simulink model "mdl_closed_loop_mpc"  (R2025a)
settings: Solver=VariableStepAuto  StartTime=0.0  StopTime=40  RelTol=1e-3
undefined symbols (not defined in the file or in its folder): coreData, onlineData
settings Model: Creator=hoshino  LastModifiedBy=root
settings ModelReferenceCC: EnableRefExpFcnMdlSchedulingChecks=on
settings RTWCC: GPUComputeCapability=3.5

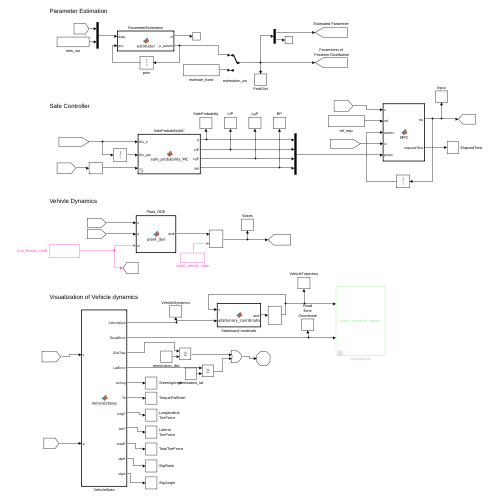
[thumbnail: Simulink's stored preview of the top-level diagram]
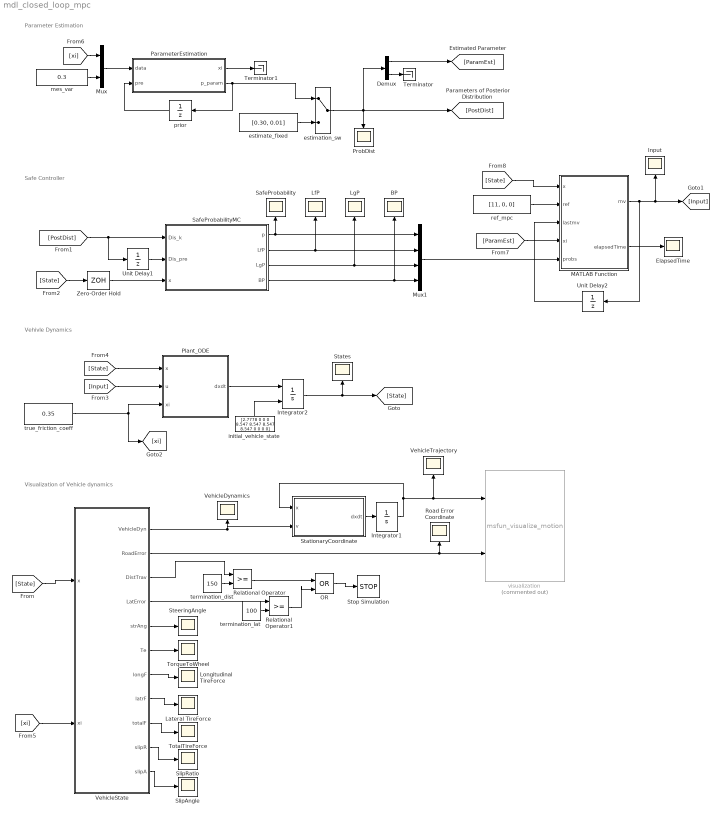
== system mdl_closed_loop_mpc ==
  note: Visualization of Vehicle dynamics
  note: Parameter Estimation
  note: Safe Controller
  note: Vehivle Dynamics
  BP : Scope
      settings: ActiveDisplayYMinimum=-0.13375  ActiveDisplayYMaximum=0.10375  DataLoggingVariableName=BP
  Demux : Demux  Outputs=2
  ElapsedTime : Scope
      settings: SampleTime=0.1  ActiveDisplayYMinimum=-0.96659  ActiveDisplayYMaximum=0.91637  DataLoggingVariableName=ElapsedTime
  Input : Scope
      settings: ActiveDisplayYMinimum=-0.96659  ActiveDisplayYMaximum=0.91637  DataLoggingVariableName=Input
  Integrator1 : Integrator  InitialCondition=[0; 0; 0]
  Integrator2 : Integrator  InitialConditionSource=external
  Lateral TireForce : Scope
      settings: ActiveDisplayYMinimum=-924.98438  ActiveDisplayYMaximum=1900.60095
  LfP : Scope
      settings: ActiveDisplayYMinimum=-5.7375  ActiveDisplayYMaximum=1.6375  DataLoggingVariableName=LfP
  LgP : Scope
      settings: ActiveDisplayYMinimum=-2.175  ActiveDisplayYMaximum=0.575  DataLoggingVariableName=LgP
  Longitudinal TireForce : Scope
      settings: ActiveDisplayYMinimum=-313.11882  ActiveDisplayYMaximum=375.42257
  MATLAB Function : MATLAB Function  TreatAsAtomicUnit=on
  Mux : Mux  Inputs=2
  Mux1 : Mux
  OR : Logic  Operator=OR  IconShape=distinctive  AllPortsSameDT=off  OutDataTypeStr=boolean
  ParameterEstimation : MATLAB Function  TreatAsAtomicUnit=on
  Plant_ODE : MATLAB Function  TreatAsAtomicUnit=on
  ProbDist : Scope
      settings: ActiveDisplayYMinimum=-0.11139  ActiveDisplayYMaximum=1.00583  DataLoggingVariableName=ProbDist
  Relational Operator : RelationalOperator  OutDataTypeStr=boolean  RndMeth=Simplest  InputSameDT=off
  Relational Operator1 : RelationalOperator  OutDataTypeStr=boolean  RndMeth=Simplest  InputSameDT=off
  Road Error Coordinate : Scope
      settings: ActiveDisplayYMinimum=-5E-5  ActiveDisplayYMaximum=0.0002  DataLoggingVariableName=ScopeData3
  SafeProbability : Scope
      settings: ActiveDisplayYMinimum=-0.125  ActiveDisplayYMaximum=1.125  DataLoggingVariableName=SafeProb
  SafeProbabilityMC : MATLAB Function  TreatAsAtomicUnit=on  mask{snum=100, dt=1.5, horizon=5, emax=10}
  SlipAngle : Scope
      settings: ActiveDisplayYMinimum=-0.25893  ActiveDisplayYMaximum=0.1231  DataLoggingVariableName=slipA
  SlipRatio : Scope
      settings: ActiveDisplayYMinimum=-0.0048  ActiveDisplayYMaximum=0.00922  DataLoggingVariableName=slipR
  States : Scope
      settings: SampleTime=0.1  ActiveDisplayYMinimum=-179.2878  ActiveDisplayYMaximum=230.07424  DataLoggingVariableName=State
  StationaryCoordinate : MATLAB Function  TreatAsAtomicUnit=on
  SteeringAngle : Scope
      settings: ActiveDisplayYMinimum=-0.32134275248447025  ActiveDisplayYMaximum=0.39116625122994469
  Stop Simulation : Stop
  Terminator : Terminator
  Terminator1 : Terminator
  TorqueToWheel : Scope
      settings: ActiveDisplayYMinimum=-256.25579  ActiveDisplayYMaximum=271.06293  DataLoggingVariableName=ScopeData2
  TotalTireForce : Scope
      settings: ActiveDisplayYMinimum=-70.03908  ActiveDisplayYMaximum=630.35171  DataLoggingVariableName=TireForce
  Unit Delay1 : UnitDelay  SampleTime=-1  HasFrameUpgradeWarning=on
  Unit Delay2 : UnitDelay  SampleTime=-1  HasFrameUpgradeWarning=on
  VehicleDynamics : Scope
      settings: ActiveDisplayYMinimum=-0.80591  ActiveDisplayYMaximum=6.57776  DataLoggingVariableName=ScopeData2
  VehicleState : MATLAB Function  TreatAsAtomicUnit=on
  VehicleTrajectory : Scope
      settings: SampleTime=0.1  ActiveDisplayYMinimum=81.20316  ActiveDisplayYMaximum=88.79585  DataLoggingVariableName=Trajectory
  Zero-Order Hold : ZeroOrderHold  SampleTime=0.1
  estimate_fixed : Constant  Value=[0.30, 0.01]
  estimation_sw : ManualSwitch
  initial_vehicle_state : Constant  Value="[2.7778           0           0           0       8.547       8.547       8.547       8.547           0           0           0           0]"
  mes_var : Constant  Value=0.3
  prior : UnitDelay  InitialCondition=[0.9 0.3]  SampleTime=-1  HasFrameUpgradeWarning=on
  ref_mpc : Constant  Value=[11, 0, 0]  VectorParams1D=off
  termination_dist : Constant  Value=150
  termination_lat : Constant  Value=100
  true_friction_coeff : Constant  Value=0.35
  visualization : M-S-Function  Commented=on  FunctionName=msfun_visualize_motion
  wires:
  Integrator2/1 -> States/1, [State]
  VehicleState/1(VehicleDyn) -> StationaryCoordinate/2(v), VehicleDynamics/1
  Integrator1/1 -> VehicleTrajectory/1, visualization/1, StationaryCoordinate/1(x)
  StationaryCoordinate/1(dxdt) -> Integrator1/1
  Plant_ODE/1(dxdt) -> Integrator2/1
  initial_vehicle_state/1 -> Integrator2/2
  true_friction_coeff/1 -> Plant_ODE/3(xi), [xi]
  [State] -> VehicleState/1(x)
  MATLAB Function/1(mv) -> Unit Delay2/1, Input/1, [Input]
  ParameterEstimation/2(p_param) -> estimation_sw/1, prior/1
  prior/1 -> ParameterEstimation/2(pre)
  ParameterEstimation/1(xi) -> Terminator1/1
  [State] -> Zero-Order Hold/1
  SafeProbabilityMC/1(p) -> SafeProbability/1, Mux1/1
  Zero-Order Hold/1 -> SafeProbabilityMC/3(x)
  [Input] -> Plant_ODE/2(u)
  [State] -> Plant_ODE/1(x)
  VehicleState/7(longF) -> Longitudinal TireForce/1
  SafeProbabilityMC/4(BP) -> Mux1/4, BP/1
  [PostDist] -> Unit Delay1/1, SafeProbabilityMC/1(Dis_k)
  Unit Delay1/1 -> SafeProbabilityMC/2(Dis_pre)
  VehicleState/9(totalF) -> TotalTireForce/1
  SafeProbabilityMC/2(LfP) -> LfP/1, Mux1/2
  SafeProbabilityMC/3(LgP) -> LgP/1, Mux1/3
  VehicleState/8(latrF) -> Lateral TireForce/1
  [xi] -> VehicleState/2(xi)
  VehicleState/10(slipR) -> SlipRatio/1
  VehicleState/11(slipA) -> SlipAngle/1
  VehicleState/2(RoadError) -> visualization/2, Road Error Coordinate/1
  Mux/1 -> ParameterEstimation/1(data)
  VehicleState/5(strAng) -> SteeringAngle/1
  VehicleState/6(Te) -> TorqueToWheel/1
  Relational Operator/1 -> OR/1
  VehicleState/3(DistTrav) -> Relational Operator/1
  termination_dist/1 -> Relational Operator/2
  estimation_sw/1 -> Demux/1, ProbDist/1, [PostDist]
  estimate_fixed/1 -> estimation_sw/2
  mes_var/1 -> Mux/2
  [xi] -> Mux/1
  OR/1 -> Stop Simulation/1
  VehicleState/4(LatError) -> Relational Operator1/1
  termination_lat/1 -> Relational Operator1/2
  Relational Operator1/1 -> OR/2
  Unit Delay2/1 -> MATLAB Function/3(lastmv)
  ref_mpc/1 -> MATLAB Function/2(ref)
  Demux/1 -> [ParamEst]
  Demux/2 -> Terminator/1
  [ParamEst] -> MATLAB Function/4(xi)
  [State] -> MATLAB Function/1(x)
  Mux1/1 -> MATLAB Function/5(probs)
  MATLAB Function/2(elapsedTime) -> ElapsedTime/1

== matlab function mdl_closed_loop_mpc/StationaryCoordinate ==
  data: x input; v input; dxdt output
function dxdt = stationary_coordinate(x,v)

    % current coordinate
    %X   = x(1); 
    %Y   = x(2); 
    Psi = x(3);
    
    % velocities
    Vx = v(1);
    Vy = v(2);
    r  = v(3);
    
    dxdt = zeros(size(x));
    dxdt(1) = Vx*cos(Psi) - Vy*sin(Psi);
    dxdt(2) = Vy*cos(Psi) + Vx*sin(Psi);
    dxdt(3) = r;

== matlab function mdl_closed_loop_mpc/ParameterEstimation ==
  data: xi output; data input; p_param output; pre input
function [xi, p_param] = estimator(data, pre)

    p_param = mfun_estimator(data, pre);
    xi = p_param(1);

== matlab function mdl_closed_loop_mpc/SafeProbabilityMC ==
  settings: updateMethod=DISCRETE
  data: Dis_k input; Dis_pre input; p output double size=1; x input; dt parameter; snum parameter; horizon parameter; LfP output double size=1; LgP output double size=[1,2]; BP output double size=1; emax parameter
function [p,LfP, LgP, BP] = safe_probability_MC(Dis_k,Dis_pre, x,dt,snum,horizon,emax)

    if Dis_pre == 0
        Dis_pre = Dis_k;
    end
    
    [p, LfP, LgP, BP] = mfun_safe_probability_MC(x, Dis_k,Dis_pre, dt,snum,horizon,emax);

== matlab function mdl_closed_loop_mpc/MATLAB Function ==
  settings: updateMethod=DISCRETE  sampleTime=0.2
  data: x input; mv output; ref input; lastmv input; xi input; probs input; onlineData parameter; coreData parameter; elapsedTime output
function [mv, elapsedTime] = MPC(x, ref, lastmv, xi, probs, onlineData, coreData)

    data = onlineData;
    data.ref = ref; %[40*1000/3600 0 0];
    data.Parameters = { xi, probs }; 

    coder.extrinsic("fun_mpc_controller");
    mv = [0;0];
    tic
    mv = fun_mpc_controller(coreData, x, lastmv, data);
    elapsedTime = toc;
    %disp(elapsedTime)

== matlab function mdl_closed_loop_mpc/VehicleState ==
  data: x input; VehicleDyn output; RoadError output; DistTrav output; LatError output; strAng output; Te output; longF output; latrF output; totalF output; xi input; slipR output; slipA output
function [VehicleDyn, RoadError, DistTrav, LatError, strAng, Te, longF, latrF, totalF, slipR, slipA]   = VehicleStates(x, xi)

% Vehicle dyanmics
VehicleDyn = x(1:3);

% Distance traveled
DistTrav = x(10);

% Lateral error
LatError = abs(x(11));


% Road error coordinate
RoadError = x(11:12);

% Steering and Input trque
strAng = x(4);
Te     = x(9);

% Tire forces
tireF = lugre_tireF(x, xi); 
longF = tireF(:,1); % longitudinal force
latrF = tireF(:,2); % lateral force
Ftfl = sqrt( tireF(1,1)^2 + tireF(1,2)^2);
Ftfr = sqrt( tireF(2,1)^2 + tireF(2,2)^2);
Ftrl = sqrt( tireF(3,1)^2 + tireF(3,2)^2);
Ftrr = sqrt( tireF(4,1)^2 + tireF(4,2)^2);
totalF = [Ftfl Ftfr Ftrl Ftrr]; % total force

% Slip ratio and Slip angle
slipR = lugre_slipR(x);
slipA = lugre_slipA(x);

== matlab function mdl_closed_loop_mpc/Plant_ODE ==
  data: x input; u input; dxdt output; xi input
function dxdt = plant_dyn(x,u,xi)

 dxdt = fun_f(x,xi) + fun_g(x)* u;

%   dxdt = suppl_mdl_vehicle_lateral(x,u);
